simulink model "PowerTransmissionModel"  (R2024a)
settings: Solver=VariableStepAuto  StartTime=0.0  StopTime=1  RelTol=1e-3
libraries: ee_lib x10, fl_lib x7, nesl_utility x3
settings Model: Creator=pvenupra  LastModifiedBy=pvenupra

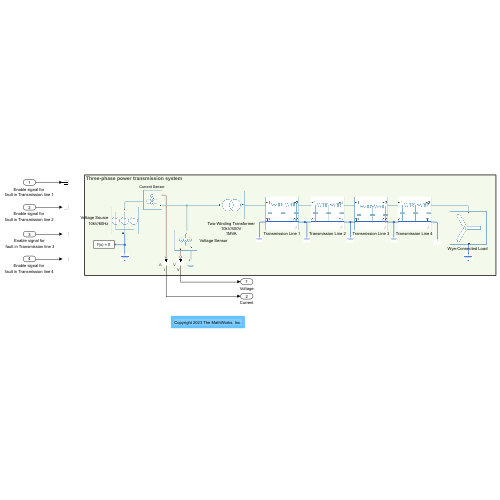
[thumbnail: Simulink's stored preview of the top-level diagram]
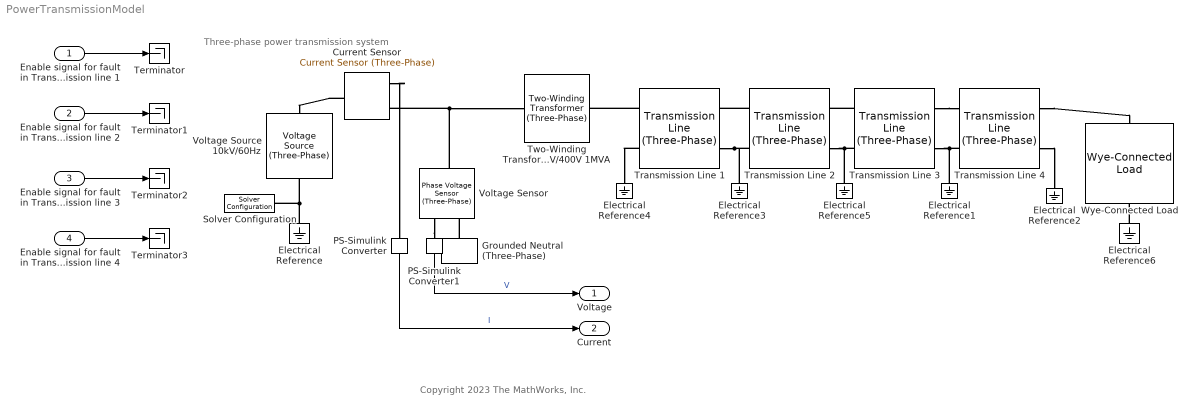
== system PowerTransmissionModel ==
  note: Copyright 2023 The MathWorks, Inc.
  note: Three-phase power transmission system
  Enable signal for fault in Transmission line 1 : Inport  SampleTime=0.025
  Enable signal for fault in Transmission line 2 : Inport  Port=2  SampleTime=0.025
  Enable signal for fault in Transmission line 3 : Inport  Port=3  SampleTime=0.025
  Enable signal for fault in Transmission line 4 : Inport  Port=4  SampleTime=0.025
  "Current Sensor " : ee_lib/Sensors & Transducers/Current Sensor (Three-Phase)
  Electrical Reference{,1..6} (7 alike) : fl_lib/Electrical/Electrical Elements/Electrical Reference
  Grounded Neutral (Three-Phase) : ee_lib/Connectors & References/Grounded Neutral (Three-Phase)
  PS-Simulink Converter : nesl_utility/PS-Simulink Converter  PhysicalDomain=network_engine_domain  SubClassName=ps_output  LeftPortType=input  RightPortType=output  PseudoPeriodic=off  Frequencies=[]  VectorFormat=1-D array  Unit=A  AffineConversion=off
  PS-Simulink Converter1 : nesl_utility/PS-Simulink Converter  PhysicalDomain=network_engine_domain  SubClassName=ps_output  LeftPortType=input  RightPortType=output  PseudoPeriodic=off  Frequencies=[]  VectorFormat=1-D array  Unit=V  AffineConversion=off
  Solver Configuration : nesl_utility/Solver Configuration  PhysicalDomain=network_engine_domain  SubClassName=solver  LeftPortType=input  RightPortType=generic  Tones=[]  Harmonics=[]  SimulateNoise=off  Profile=off  UseLocalSampling=off  EnableSwitchedLinearOptims=on  FrequencyDomain=off  UseCCode=off  RelTol=0.001  AbsTol=1e-06  MinStep=1e-09  ToWorkspace=off  RevertToSquareIcSolve=off  NumHomotopyIterations=100  PhasorMode=off  PhasorModeNumHarmonics=1  ConsistencySolver=NEWTON_FTOL  IndexReductionMethod=DerivativeReplacement  DoDC=off  ResidualTolerance=1e-09  ConsistencyTolSource=GLOBAL  ConsistencyAbsTol=0.001  ConsistencyRelTol=0.001  ConsistencyTolFactor=0.001  UseLocalSolver=on  LocalSolverChoice=NE_BACKWARD_EULER_ADVANCER  ResolveIndetEquations=on  FunctionEvalNumThread=1  LocalSolverSampleTime=1e-4  DoFixedCost=on  MaxNonlinIter=3  MaxModeIter=2  ComputeImpulses=off  ImpulseIterations=2  LinearAlgebra=auto  LinearAlgebraNumThread=0  EquationFormulation=NE_TIME_EF  DelaysMemoryBudget=1024  AutomaticFiltering=on  FilteringTimeConstant=0.001  PartitionStorageMethod=AS_NEEDED  PartitionMemoryBudget=1024  PartitionMethod=FAST  MultibodyUseLocalSolver=off  MultibodyLocalSolverChoice=ODE1  MultibodyLocalSolverSampleTime=0.001
  Terminator{,1..3} (4 alike) : Terminator
  Transmission Line {1..4} (4 alike) : ee_lib/Passive/Lines/Transmission Line (Three-Phase)  length=0.1 km  freq=60 Hz  R=.02 Ohm/km  L=0.5 mH/km  M=0.1 mH/km  Cl=0.3 uF/km  Cg=.1 uF/km  Rm=0 Ohm/km  ModelTwoSections=ee.enum.enable.yes  N=1  InterfacePosition=0.05 km  N1sec=1  N2sec=1  Access_ground=ee.enum.enable.no  R_parasitic=1e-6 Ohm  G_parasitic=1e-6 1/Ohm  EnableFault=false  fault_type_option=ee.enum.fault_type_option.ag  R_pn_fault=1e-3 Ohm  R_ng_fault=1e-3 Ohm  unfaulted_G_parasitic=1e-6 1/Ohm
      settings: InternalSimscapePortConfiguration="{\"Bottom\":[],\"Left\":[{\"id\":\"N1\",\"label\":\"~1\",\"type\":\"foundation.electrical.three_phase\"},{\"id\":\"g1\",\"label\":\"g1\",\"type\":\"foundation.electrical.electrical\"}],\"Right\":[{\"id\":\"N2\",\"label\":\"~2\",\"type\":\"foundation.electrical.three_phase\"},{\"id\":\"g2\",\"label\":\"g2\",\"type\":\"foundation.electrical.electrical\"}],\"Top\":[]}"
  Two-Winding Transformer 10kV/400V 1MVA : ee_lib/Passive/Transformers/Two-Winding Transformer (Three-Phase)  SRated=1e6 A*V  FRated=60 Hz  Winding1Connection=ee.enum.windingconnection.Yg  VRated1=10000 V  Winding2Connection=ee.enum.windingconnection.Yg  VRated2=400 V  CoreType=ee.enum.coretype.fivelimb  pu_Rw1=0.002  pu_Rw2=0.002  leakage_reactance_option=ee.enum.transformer_leakage.exclude  pu_Xl1=0.05  pu_Xl2=0.05  magnetizing_resistance_option=ee.enum.transformer_magnetizingResistance.include  pu_Rm=500  magnetizing_reactance_option=ee.enum.transformer_magnetizingReactance.include  saturation_option=ee.enum.transformer_saturation.exclude  pu_Xm=500  current_data=[0, .002, 1, 2]  magnetic_flux_data=[0, 1.2, 1.5, 1.51]  pu_X0=0.5  i1_specify=off  i1_priority=None  i1=[0, 0, 0] A  i1_nominal_specify=off  i1_nominal_unit=A  i1_nominal_value=1  i2_specify=off  i2_priority=None  i2=[0, 0, 0] A  i2_nominal_specify=off  i2_nominal_unit=A  i2_nominal_value=1  phi_specify=off  phi_priority=None  phi=[0, 0, 0]  phi_nominal_specify=off  phi_nominal_unit=1  phi_nominal_value=1  power_dissipated_specify=off  power_dissipated_priority=None  power_dissipated=0 W  power_dissipated_nominal_specify=off  power_dissipated_nominal_unit=W  power_dissipated_nominal_value=1
      settings: InternalSimscapePortConfiguration="{\"Bottom\":[],\"Left\":[{\"id\":\"N1\",\"label\":\"~1\",\"type\":\"foundation.electrical.three_phase\"}],\"Right\":[{\"id\":\"N2\",\"label\":\"~2\",\"type\":\"foundation.electrical.three_phase\"}],\"Top\":[]}"
  Voltage Sensor : ee_lib/Sensors & Transducers/Phase Voltage Sensor (Three-Phase)
  Voltage Source 10kV/60Hz : ee_lib/Sources/Voltage Source (Three-Phase)  vline_rms=10000 V  shift=0 deg  freq=60 Hz  impedance_option=1  SShortCircuit=10e6 A*V  XR=7  R=0.01 Ohm  L=3.97e-4 H  harmonic_option=0  harmonic_orders=[5, 7, 11, 13]  harmonic_ratios=[.1, .1, .1, .1]  G_parasitic=0 1/Ohm  I_specify=off  I_priority=None  I=[0, 0, 0] A  I_nominal_specify=off  I_nominal_unit=A  I_nominal_value=1
  "Wye-Connected Load " : ee_lib/Passive/RLC Assemblies/Wye-Connected Load  parameterization=ee.enum.rlc.parameterization.ratedpower  component_structure=ee.enum.rlc.structure.R  component_structure_PQ=ee.enum.rlc.structure.SeriesRL  R=1 Ohm  L=1e-3 H  C=1e-6 F  VRated=400 V  FRated=60 Hz  P=4e5 W  Qpos=1e5 A*V  Qneg=-1e2 A*V  R_parasitic=0 Ohm  G_parasitic=0 1/Ohm  R_parasitic_PQ=0 Ohm  G_parasitic_PQ=0 1/Ohm  Vmag0=400 V  Vang0=0 deg  Freq0=60 Hz  IL_specify=off  IL_priority=High  IL=[0, 0, 0] A  IL_nominal_specify=off  IL_nominal_unit=A  IL_nominal_value=1  VC_specify=off  VC_priority=High  VC=[0, 0, 0] V  VC_nominal_specify=off  VC_nominal_unit=V  VC_nominal_value=1
  Voltage : Outport
  Current : Outport  Port=2
  wires:
  PS-Simulink Converter1/1 -> Voltage/1  "V"
  PS-Simulink Converter/1 -> Current/1  "I"
  Enable signal for fault in Transmission line 1/1 -> Terminator/1
  Enable signal for fault in Transmission line 2/1 -> Terminator1/1
  Enable signal for fault in Transmission line 3/1 -> Terminator2/1
  Enable signal for fault in Transmission line 4/1 -> Terminator3/1
  connections:
  Electrical Reference/LConn1 -- Voltage Source 10kV/60Hz/LConn1 -- Solver Configuration/RConn1
  "Current Sensor "/LConn1 -- Voltage Source 10kV/60Hz/RConn1
  Transmission Line 1/LConn1 -- Two-Winding Transformer 10kV/400V 1MVA/RConn1
  Transmission Line 1/LConn2 -- Electrical Reference4/LConn1
  Transmission Line 2/LConn1 -- Transmission Line 1/RConn1
  Electrical Reference3/LConn1 -- Transmission Line 2/LConn2 -- Transmission Line 1/RConn2
  Transmission Line 3/LConn1 -- Transmission Line 2/RConn1
  Electrical Reference5/LConn1 -- Transmission Line 3/LConn2 -- Transmission Line 2/RConn2
  Transmission Line 3/RConn1 -- Transmission Line 4/LConn1
  Electrical Reference1/LConn1 -- Transmission Line 3/RConn2 -- Transmission Line 4/LConn2
  Transmission Line 4/RConn2 -- Electrical Reference2/LConn1
  "Current Sensor "/RConn1 -- PS-Simulink Converter/LConn1
  Voltage Sensor/RConn1 -- PS-Simulink Converter1/LConn1
  Electrical Reference6/LConn1 -- "Wye-Connected Load "/RConn1
  Transmission Line 4/RConn1 -- "Wye-Connected Load "/LConn1
  Voltage Sensor/LConn1 -- Two-Winding Transformer 10kV/400V 1MVA/LConn1 -- "Current Sensor "/RConn2
  Grounded Neutral (Three-Phase)/LConn1 -- Voltage Sensor/RConn2
